simulink model "bol1_ejer4_grafica"  (R2021a)
settings: Solver=VariableStepAuto  StartTime=0.0  StopTime=10.0  RelTol=1e-3
settings Model: Creator=andrea  LastModifiedBy=andrea

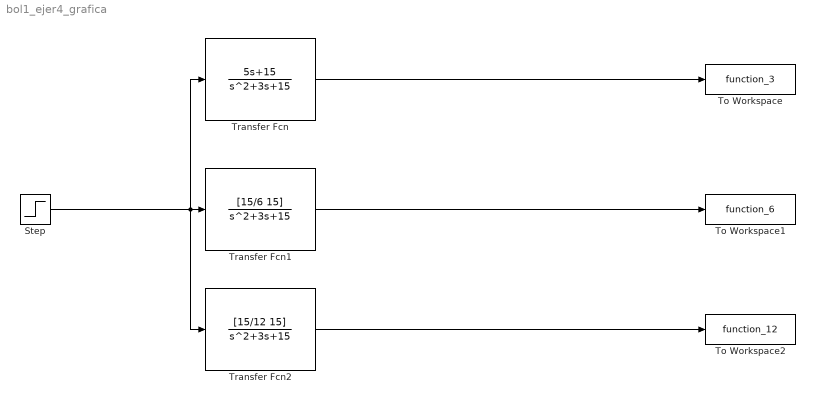
== system bol1_ejer4_grafica ==
  Step : Step  SampleTime=0
  To Workspace : ToWorkspace  VariableName=function_3  SampleTime=-1
  To Workspace1 : ToWorkspace  VariableName=function_6  SampleTime=-1
  To Workspace2 : ToWorkspace  VariableName=function_12  SampleTime=-1
  Transfer Fcn : TransferFcn  Numerator=[5 15]  Denominator=[1 3 15]
  Transfer Fcn1 : TransferFcn  Numerator=[15/6 15]  Denominator=[1 3 15]
  Transfer Fcn2 : TransferFcn  Numerator=[15/12 15]  Denominator=[1 3 15]
  wires:
  Step/1 -> Transfer Fcn/1, Transfer Fcn2/1, Transfer Fcn1/1
  Transfer Fcn1/1 -> To Workspace1/1
  Transfer Fcn2/1 -> To Workspace2/1
  Transfer Fcn/1 -> To Workspace/1
